simulink model "SchemaControlloDecentralizzatoSmartSixR2013a"  (Simulink 8.4)
settings: Solver=ode23  StartTime=0.0  StopTime=t(end)+Tf  FixedStep=T  RelTol=1e-3
PreLoadFcn:
  | initFunction
InitFcn:
  | initFunction
StopFcn:
  | figure
  | subplot(31,1)
  | plot(err_q.data(1:50))
  | subplot(312)
  | plot(err_dq.data(1:50))
  | subplot(313)
  | plot(err_ddq.data(1:50))
values from neighbouring files (symbols this model uses):
  FM = Kr^-1*Fv*Kr^-1    [ControlloreUnico.m]    (also in SimulazioneLsim.m = Kr^-1*Fv_att*Kr^-1; initFunction.m; initFunctionIm.m)
  Im = Kr^-1*Bconst*Kr^-1    [initFunction.m]    (also in initFunctionIm.m)
  KCA = diag([(-W(1,1)^2 + KM(1,1)*XR(1,1))/(KM(1,1)*KTA(1,1)*W(1,1)^2),             (-W(2,2)^2 + KM(2,2)*XR(2,2))/(KM(2,2)*KTA(2,2)*W(2,2)^2),             (-W(3,3)^2 + KM(3,3)*XR(3,3))/(KM(3,3)*KTA(3,3)*W(3,3)^2),             (-W(4,4)^2 + KM(4,4)*XR(4,4))/(KM(4,4)*KTA(4,4)*W(4,4)^2),             (-W(5,5)^2 + KM(5,5)*XR(5,5))/(KM(5,5)*KTA(5,5)*W(5,5)^2),             (-W(6,6)^2 + KM(6,6)*XR(6,6))/(KM(6,6)* ...(+20 chars)    [DesignControllersAcceleration_6.m]    (also in DesignControllersAcceleration_7.m; DiscreteControllersAcceleration_7.m)
  KCP = diag([(KTV(1,1)*W(1,1))/(2*KTP(1,1)*Z(1,1)),             (KTV(2,2)*W(2,2))/(2*KTP(2,2)*Z(2,2)),             (KTV(3,3)*W(3,3))/(2*KTP(3,3)*Z(3,3)),             (KTV(4,4)*W(4,4))/(2*KTP(4,4)*Z(4,4)),             (KTV(5,5)*W(5,5))/(2*KTP(5,5)*Z(5,5)),             (KTV(6,6)*W(6,6))/(2*KTP(6,6)*Z(6,6))])    [DesignControllersAcceleration_6.m]    (also in DesignControllersAcceleration_7.m; DesignControllersVelocity_6.m; DiscreteControllersAcceleration_7.m; DiscreteDesignControllersVelocity_6.m)
  KCV = diag([(2*KM(1,1)*KTA(1,1)*W(1,1)*XR(1,1)*Z(1,1))/(KTV(1,1)*(-W(1,1)^2 + KM(1,1)*XR(1,1))),             (2*KM(2,2)*KTA(2,2)*W(2,2)*XR(2,2)*Z(2,2))/(KTV(2,2)*(-W(2,2)^2 + KM(2,2)*XR(2,2))),             (2*KM(3,3)*KTA(3,3)*W(3,3)*XR(3,3)*Z(3,3))/(KTV(3,3)*(-W(3,3)^2 + KM(3,3)*XR(3,3))),             (2*KM(4,4)*KTA(4,4)*W(4,4)*XR(4,4)*Z(4,4))/(KTV(4,4)*(-W(4,4)^2 + KM(4,4)*XR(4,4))),             (2*KM( ...(+176 chars)    [DesignControllersAcceleration_6.m]    (also in DesignControllersAcceleration_7.m; DesignControllersVelocity_6.m = diag([(2*W(1,1)*Z(1,1))/(KM(1,1)*KTV(1,1)),             (2*W; DiscreteControllersAcceleration_7.m = diag([(rlkcv(1)*KM(1,1)*KTA(1,1)*W(1,1)*XR(1,1)*Z(1,1))/(KTV; DiscreteDesignControllersVelocity_6.m = diag([rlkcv(1)*(2*W(1,1)*Z(1,1))/(KM(1,1)*KTV(1,1)),        )
  KM = Kv^-1    [DesignControllersAcceleration_6.m]    (also in DesignControllersAcceleration_7.m; DesignControllersVelocity_6.m; DiscreteControllersAcceleration_7.m; DiscreteDesignControllersVelocity_6.m)
  KTA = diag([100 1 1 1 1 1])    [DesignControllersAcceleration_6.m]    (also in DesignControllersAcceleration_7.m = diag([1 1 1 1 1 1]); DiscreteControllersAcceleration_7.m = diag([1 1 1 1 1 1]))
  KTP = diag([9 1 1 1 1 1])    [DesignControllersAcceleration_6.m]    (also in DesignControllersAcceleration_7.m = diag([1 1 1 1 1 1]); DesignControllersVelocity_6.m = diag([1 1 1 1 1 1]); DiscreteControllersAcceleration_7.m = diag([1 1 1 1 1 1]); DiscreteDesignControllersVelocity_6.m = diag([1 1 1 1 1 1]))
  KTV = diag([4 1 1 1 1 1])    [DesignControllersAcceleration_6.m]    (also in DesignControllersAcceleration_7.m = diag([1 1 1 1 1 1]); DesignControllersVelocity_6.m = diag([1 1 1 1 1 1]); DiscreteControllersAcceleration_7.m = diag([1 1 1 1 1 1]); DiscreteDesignControllersVelocity_6.m = diag([1 1 1 1 1 1]))
  q0 = q0'    [initFunction.m]    (also in initFunctionIm.m)
  T = 0.05    [ComputeBconst_4.m]    (also in ControlloreUnico.m = 0.002; Identificazione_2.m = 0:1/F:(size(min_value,2)-1)*interval; Simulazione.m = 0.002; SimulazioneLsim.m = 0.002)
  TCA = diag([Tm(1,1) Tm(2,2) Tm(3,3) Tm(4,4) Tm(5,5) Tm(6,6)])    [DesignControllersAcceleration_6.m]    (also in DesignControllersAcceleration_7.m = diag([TM(1,1) TM(2,2) TM(3,3) TM(4,4) TM(5,5) TM(6,6)]); DiscreteControllersAcceleration_7.m = diag([TM(1,1) TM(2,2) TM(3,3) TM(4,4) TM(5,5) TM(6,6)]))
undefined symbols (not defined in the file or in its folder): Kr, Kt, Kv, La, Ra
libraries: simulink x18
(part 1 of 2)
CloseFcn:
  | rtwprivate ssgencode ModelCloseRequest ContributiCoppieComau
settings Model: Creator=Alessandro  LastModifiedBy=Leonardo  SimulationMode=accelerator  ExtModeAutoUpdateStatusClock=off  BufferReuse=off
settings DataIOCC: SaveFormat=StructureWithTime  SignalLoggingSaveFormat=Dataset
settings OptimizationCC: BlockReduction=off  BufferReuse=off  InitFltsAndDblsToZero=on
settings DebuggingCC: AlgebraicLoopMsg=none  SaveWithParameterizedLinksMsg=none  SignalResolutionControl=TryResolveAllWithWarning  SolverPrmCheckMsg=none  InheritedTsInSrcMsg=none  MultiTaskDSMMsg=warning  MultiTaskCondExecSysMsg=none  TasksWithSamePriorityMsg=none  UnconnectedInputMsg=none  UnconnectedOutputMsg=none  UnconnectedLineMsg=none  FrameProcessingCompatibilityMsg=error
settings GRTTargetCC: TargetFcnLib=ansi_tfl_tmw.mat
settings ConfigComp: CovMetricSettings=dw  CovHtmlReporting=on  CovSaveCumulativeToWorkspaceVar=on  CovSaveSingleToWorkspaceVar=on  CovModelRefEnable=Off  CovExternalEMLEnable=off

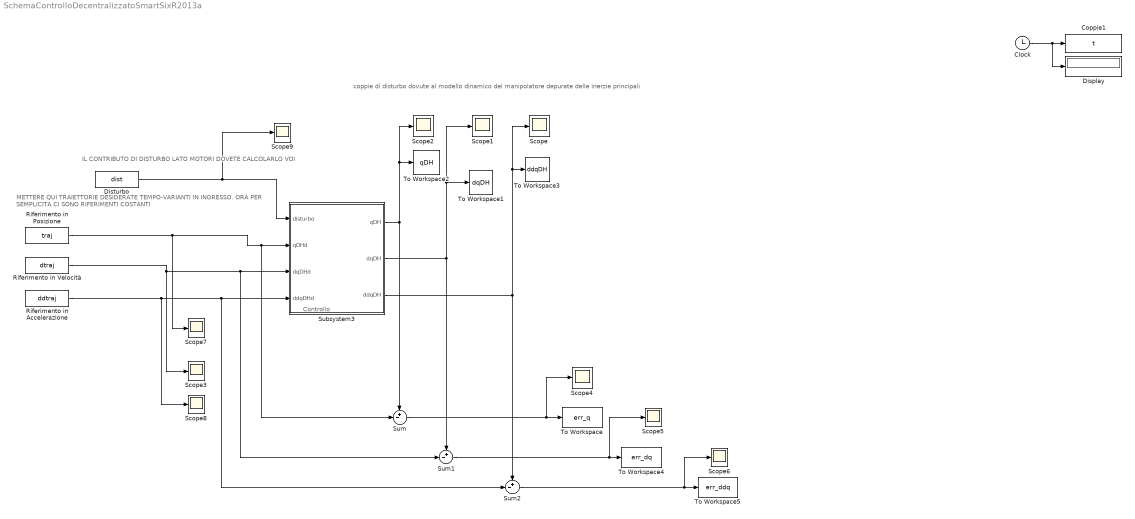
== system SchemaControlloDecentralizzatoSmartSixR2013a ==
  note: coppie di disturbo dovute al modello dinamico del manipolatore depurate delle inerzie principali
  note: Controllo
  note: METTERE QUI TRAIETTORIE DESIDERATE TEMPO-VARIANTI IN INGRESSO.
      | ORA PER SEMPLICITA CI SONO RIFERIMENTI COSTANTI
  note: IL CONTRIBUTO DI DISTURBO LATO MOTORI DOVETE CALCOLARLO VOI
  Clock : Clock
  Coppie1 : ToWorkspace  VariableName=t  SampleTime=-1
  Display : Display
  Disturbo : FromWorkspace  VariableName=dist  Interpolate=off  OutputAfterFinalValue=Holding final value
  Riferimento in Accelerazione : FromWorkspace  VariableName=ddtraj
  Riferimento in Posizione : FromWorkspace  VariableName=traj
  Riferimento in Velocità : FromWorkspace  VariableName=dtraj
  Scope{,1..9} (10 alike) : Scope
      Scope settings: TimeRange=0.4  YMin=-3427537178483172600000000000000000000000000000000000000000000000000000000000000000000000000000000000000000000000000000000000000000000000000000000000000000000000000000000000000000000000000000000000000000000000000000000000000000000000000000000000000000000000000000000000000000000000000000000000000000000.00000  YMax=6302006154523578300000000000000000000000000000000000000000000000000000000000000000000000000000000000000000000000000000000000000000000000000000000000000000000000000000000000000000000000000000000000000000000000000000000000000000000000000000000000000000000000000000000000000000000000000000000000000000000.00000
      Scope1 settings: YMin=-1.00000  YMax=1.00000
      Scope2 settings: TimeRange=0.01894736842105263  YMin=-1  YMax=1  SaveName=ScopeData2
      Scope3 settings: TimeRange=0.01894736842105263  YMin=-11.17185  YMax=11.83001  SaveName=ScopeData4
      Scope4 settings: TimeRange=5.918947368421053  YMin=-0.04  YMax=0.01
      Scope5 settings: TimeRange=5.018947368421053  YMin=-0.05  YMax=0.04  SaveName=ScopeData3
      Scope6 settings: TimeRange=1.018947368421053  YMin=-8  YMax=10  SaveName=ScopeData6
      Scope7 settings: TimeRange=0.01894736842105263  YMin=-1  YMax=1  SaveName=ScopeData2
      Scope8 settings: TimeRange=0.01894736842105263  YMin=-11.17185  YMax=11.83001  SaveName=ScopeData5
      Scope9 settings: TimeRange=0.01894736842105263  YMin=-1  YMax=1  SaveName=ScopeData7
  Subsystem3 : Subsystem
      mask Display:
      | disp('Controllo');
      | port_label('input', 1, 'disturbo');
      | port_label('input', 2, 'qDHd');
      | port_label('input', 3, 'dqDHd');
      | port_label('output', 1, 'qDH');
      | port_label('output', 2, 'dqDH');
      | port_label('output', 3, 'ddqDH');
  Sum : Sum  Inputs=+-|
  Sum1 : Sum  Inputs=+-|
  Sum2 : Sum  Inputs=+-|
  To Workspace : ToWorkspace  VariableName=err_q  SaveFormat=Timeseries  SampleTime=-1
  To Workspace1 : ToWorkspace  VariableName=dqDH  SampleTime=-1
  To Workspace2 : ToWorkspace  VariableName=qDH  SampleTime=-1
  To Workspace3 : ToWorkspace  VariableName=ddqDH  SampleTime=-1
  To Workspace4 : ToWorkspace  VariableName=err_dq  SaveFormat=Timeseries  SampleTime=-1
  To Workspace5 : ToWorkspace  VariableName=err_ddq  SaveFormat=Timeseries  SampleTime=-1
  wires:
  Clock/1 -> Coppie1/1, Display/1
  Subsystem3/2(dqDH) -> Sum1/1, To Workspace1/1, Scope1/1
  Subsystem3/1(qDH) -> To Workspace2/1, Scope2/1, Sum/1
  Subsystem3/3(ddqDH) -> Sum2/1, To Workspace3/1, Scope/1
  Riferimento in Velocità/1 -> Scope3/1, Sum1/2, Subsystem3/3(dqDHd)
  Riferimento in Accelerazione/1 -> Scope8/1, Sum2/2, Subsystem3/4(ddqDHd)
  Riferimento in Posizione/1 -> Scope7/1, Sum/2, Subsystem3/2(qDHd)
  Disturbo/1 -> Scope9/1, Subsystem3/1(disturbo)
  Sum/1 -> Scope4/1, To Workspace/1
  Sum1/1 -> Scope5/1, To Workspace4/1
  Sum2/1 -> Scope6/1, To Workspace5/1

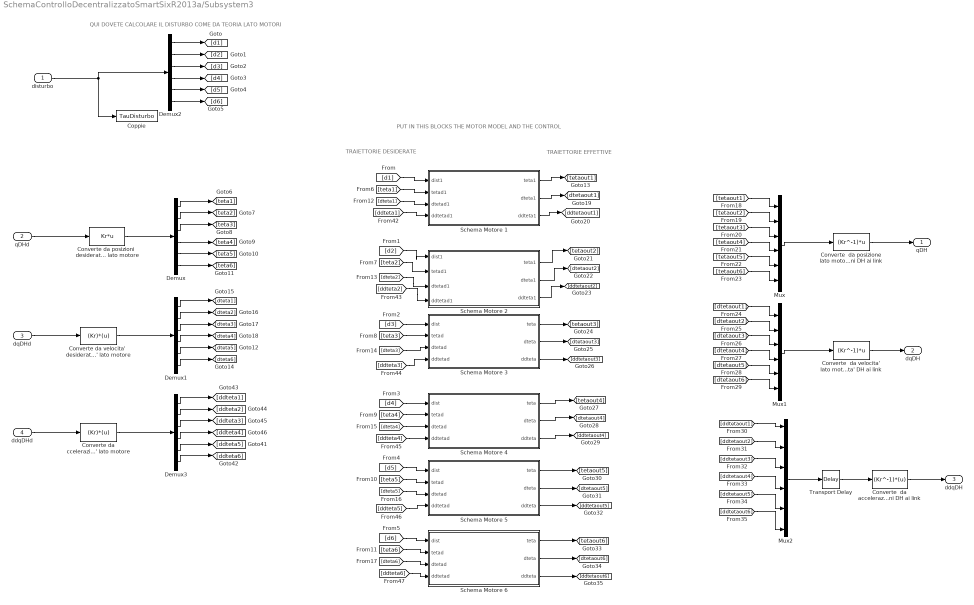
== system SchemaControlloDecentralizzatoSmartSixR2013a/Subsystem3 ==
  note: PUT IN THIS BLOCKS THE MOTOR MODEL AND THE CONTROL
  note: TRAIETTORIE DESIDERATE
  note: TRAIETTORIE EFFETTIVE
  note: QUI DOVETE CALCOLARE IL DISTURBO COME DA TEORIA LATO MOTORI
  disturbo : Inport
  qDHd : Inport  Port=2
  dqDHd : Inport  Port=3
  ddqDHd : Inport  Port=4
  Converte  da accelerazioni lato motore  ad accelerazioni DH ai link : MATLABFcn  MATLABFcn=(Kr^-1)*(u)
  "Converte  da posizione lato motore a  posizioni DH ai link " : MATLABFcn  MATLABFcn=(Kr^-1)*u
  "Converte  da velocita' lato motore  a velocita' DH ai link " : MATLABFcn  MATLABFcn=(Kr^-1)*u
  Converte da ccelerazioni  desiderate DH ai link  in velocita' lato motore : MATLABFcn  MATLABFcn=(Kr)*(u)
  "Converte da posizioni  desiderate DH ai link  in posizione lato motore " : MATLABFcn  MATLABFcn=Kr*u
  "Converte da velocita'  desiderate DH ai link  in velocita' lato motore " : MATLABFcn  MATLABFcn=(Kr)*(u)
  Coppie : ToWorkspace  VariableName=TauDisturbo  SampleTime=-1
  Demux{,1..3} (4 alike) : Demux  Outputs=6
  Mux : Mux  Inputs=6
  Mux1 : Mux  Inputs=6
  Mux2 : Mux  Inputs=6
  Schema Motore 1 : Subsystem  mask{i=1}
  Schema Motore 2 : Subsystem  mask{i=2}
  Schema Motore 3 : Subsystem  mask{i=3}
  Schema Motore 4 : Subsystem  mask{i=4}
  Schema Motore 5 : Subsystem  mask{i=5}
  Schema Motore 6 : Subsystem  mask{i=6}
  Transport Delay : TransportDelay  DelayTime=T
  qDH : Outport
  dqDH : Outport  Port=2
  ddqDH : Outport  Port=3
  wires:
  qDHd/1 -> "Converte da posizioni  desiderate DH ai link  in posizione lato motore "/1
  dqDHd/1 -> "Converte da velocita'  desiderate DH ai link  in velocita' lato motore "/1
  "Converte  da velocita' lato motore  a velocita' DH ai link "/1 -> dqDH/1
  Converte  da accelerazioni lato motore  ad accelerazioni DH ai link/1 -> ddqDH/1
  "Converte da posizioni  desiderate DH ai link  in posizione lato motore "/1 -> Demux/1
  disturbo/1 -> Coppie/1, Demux2/1
  "Converte  da posizione lato motore a  posizioni DH ai link "/1 -> qDH/1
  Mux/1 -> "Converte  da posizione lato motore a  posizioni DH ai link "/1
  Demux2/1 -> [d1]
  Demux2/2 -> [d2]
  Demux2/3 -> [d3]
  Demux2/4 -> [d4]
  Demux2/5 -> [d5]
  Demux2/6 -> [d6]
  [d3] -> Schema Motore 3/1(dist)
  Demux/1 -> [teta1]
  Demux/2 -> [teta2]
  Demux/3 -> [teta3]
  Demux/4 -> [teta4]
  Demux/5 -> [teta5]
  Demux/6 -> [teta6]
  [teta3] -> Schema Motore 3/2(tetad)
  "Converte da velocita'  desiderate DH ai link  in velocita' lato motore "/1 -> Demux1/1
  Demux1/1 -> [dteta1]
  Demux1/2 -> [dteta2]
  Demux1/3 -> [dteta3]
  Demux1/4 -> [dteta4]
  Demux1/5 -> [dteta5]
  Demux1/6 -> [dteta6]
  [dteta3] -> Schema Motore 3/3(dtetad)
  [tetaout1] -> Mux/1
  [tetaout2] -> Mux/2
  [tetaout3] -> Mux/3
  [tetaout4] -> Mux/4
  [tetaout5] -> Mux/5
  [tetaout6] -> Mux/6
  Mux1/1 -> "Converte  da velocita' lato motore  a velocita' DH ai link "/1
  [dtetaout1] -> Mux1/1
  [dtetaout2] -> Mux1/2
  [dtetaout3] -> Mux1/3
  [dtetaout4] -> Mux1/4
  [dtetaout5] -> Mux1/5
  [dtetaout6] -> Mux1/6
  [ddtetaout1] -> Mux2/1
  [ddtetaout2] -> Mux2/2
  [ddtetaout3] -> Mux2/3
  [ddtetaout4] -> Mux2/4
  [ddtetaout5] -> Mux2/5
  [ddtetaout6] -> Mux2/6
  ddqDHd/1 -> Converte da ccelerazioni  desiderate DH ai link  in velocita' lato motore/1
  Demux3/1 -> [ddteta1]
  Demux3/2 -> [ddteta2]
  Demux3/3 -> [ddteta3]
  Demux3/4 -> [ddteta4]
  Demux3/5 -> [ddteta5]
  Demux3/6 -> [ddteta6]
  Converte da ccelerazioni  desiderate DH ai link  in velocita' lato motore/1 -> Demux3/1
  Schema Motore 3/1(teta) -> [tetaout3]
  Schema Motore 3/2(dteta) -> [dtetaout3]
  Schema Motore 3/3(ddteta) -> [ddtetaout3]
  [ddteta3] -> Schema Motore 3/4(ddtetad)
  [d2] -> Schema Motore 2/1(dist1)
  [teta2] -> Schema Motore 2/2(tetad1)
  [dteta2] -> Schema Motore 2/3(dtetad1)
  [ddteta2] -> Schema Motore 2/4(ddtetad1)
  Schema Motore 2/1(teta1) -> [tetaout2]
  Schema Motore 2/2(dteta1) -> [dtetaout2]
  Schema Motore 2/3(ddteta1) -> [ddtetaout2]
  Mux2/1 -> Transport Delay/1
  Transport Delay/1 -> Converte  da accelerazioni lato motore  ad accelerazioni DH ai link/1
  [teta1] -> Schema Motore 1/2(tetad1)
  [dteta1] -> Schema Motore 1/3(dtetad1)
  [ddteta1] -> Schema Motore 1/4(ddtetad1)
  Schema Motore 1/1(teta1) -> [tetaout1]
  Schema Motore 1/2(dteta1) -> [dtetaout1]
  Schema Motore 1/3(ddteta1) -> [ddtetaout1]
  [d4] -> Schema Motore 4/1(dist)
  [teta4] -> Schema Motore 4/2(tetad)
  [dteta4] -> Schema Motore 4/3(dtetad)
  [ddteta4] -> Schema Motore 4/4(ddtetad)
  Schema Motore 4/1(teta) -> [tetaout4]
  Schema Motore 4/2(dteta) -> [dtetaout4]
  Schema Motore 4/3(ddteta) -> [ddtetaout4]
  [d5] -> Schema Motore 5/1(dist)
  [teta5] -> Schema Motore 5/2(tetad)
  [dteta5] -> Schema Motore 5/3(dtetad)
  [ddteta5] -> Schema Motore 5/4(ddtetad)
  [d6] -> Schema Motore 6/1(dist)
  [teta6] -> Schema Motore 6/2(tetad)
  [dteta6] -> Schema Motore 6/3(dtetad)
  [ddteta6] -> Schema Motore 6/4(ddtetad)
  Schema Motore 6/1(teta) -> [tetaout6]
  Schema Motore 6/2(dteta) -> [dtetaout6]
  Schema Motore 6/3(ddteta) -> [ddtetaout6]
  Schema Motore 5/3(ddteta) -> [ddtetaout5]
  Schema Motore 5/2(dteta) -> [dtetaout5]
  Schema Motore 5/1(teta) -> [tetaout5]
  [d1] -> Schema Motore 1/1(dist1)

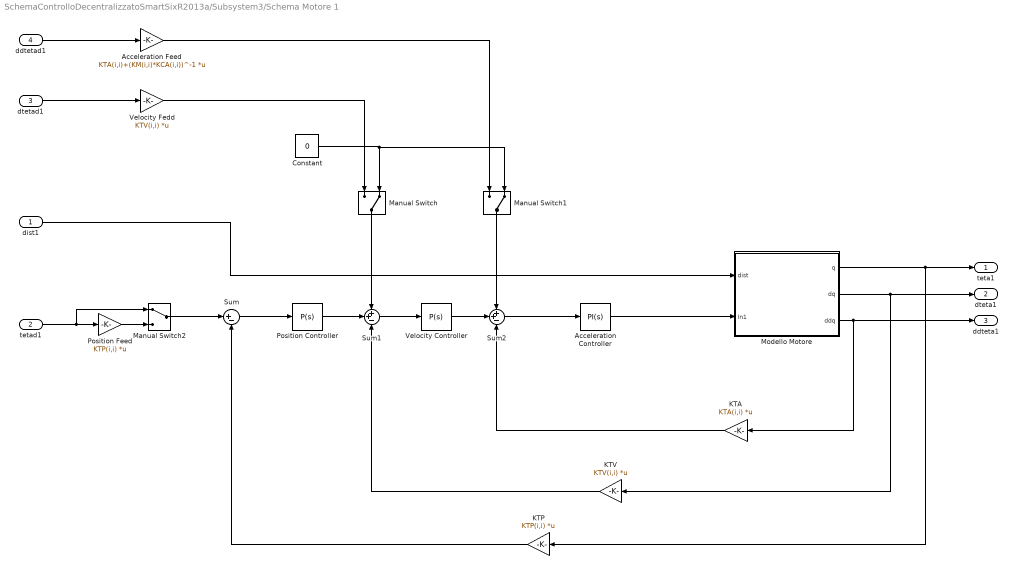
== system SchemaControlloDecentralizzatoSmartSixR2013a/Subsystem3/Schema Motore 1 ==
  dist1 : Inport  PortDimensions=1
  tetad1 : Inport  Port=2  PortDimensions=1
  dtetad1 : Inport  Port=3  PortDimensions=1
  ddtetad1 : Inport  Port=4  PortDimensions=1
  Acceleration Controller : simulink/Continuous/PID Controller  Controller=PI  TimeDomain=Continuous-time  SampleTime=-1  IntegratorMethod=Forward Euler  FilterMethod=Forward Euler  Form=Parallel  P=TCA(i,i)*KCA(i,i)  I=KCA(i,i)  D=0  N=100  InitialConditionSource=internal  InitialConditionForIntegrator=0  InitialConditionForFilter=0  ExternalReset=none  LimitOutput=off  UpperSaturationLimit=inf  LowerSaturationLimit=-inf  LinearizeAsGain=on  AntiWindupMode=none  Kb=1  TrackingMode=off  Kt=1  PParamMin=[]  PParamMax=[]  IParamMin=[]  IParamMax=[]  DParamMin=[]  DParamMax=[]  NParamMin=[]  NParamMax=[]  KbParamMin=[]  KbParamMax=[]  KtParamMin=[]  KtParamMax=[]  POutMin=[]  POutMax=[]  IOutMin=[]  IOutMax=[]  DOutMin=[]  DOutMax=[]  NOutMin=[]  NOutMax=[]  KbOutMin=[]  KbOutMax=[]  KtOutMin=[]  KtOutMax=[]  IntegratorOutMin=[]  IntegratorOutMax=[]  FilterOutMin=[]  FilterOutMax=[]  SumOutMin=[]  SumOutMax=[]  SumI1OutMin=[]  SumI1OutMax=[]  SumI2OutMin=[]  SumI2OutMax=[]  SumI3OutMin=[]  SumI3OutMax=[]  SumDOutMin=[]  SumDOutMax=[]  SaturationOutMin=[]  SaturationOutMax=[]  IntegratorContinuousStateAttributes=''  IntegratorStateMustResolveToSignalObject=off  IntegratorRTWStateStorageClass=Auto  FilterContinuousStateAttributes=''  FilterStateMustResolveToSignalObject=off  FilterRTWStateStorageClass=Auto  DifferentiatorICPrevScaledInput=0  DifferentiatorOutMin=[]  DifferentiatorOutMax=[]  UseFilter=on
  Acceleration Feed : Gain  Gain=KTA(i,i)+(KM(i,i)*KCA(i,i))^-1  Multiplication=Matrix(K*u)
  Constant : Constant  Value=0
  KTA : Gain  Gain=KTA(i,i)  Multiplication=Matrix(K*u)
  KTP : Gain  Gain=KTP(i,i)  Multiplication=Matrix(K*u)
  KTV : Gain  Gain=KTV(i,i)  Multiplication=Matrix(K*u)
  Manual Switch : ManualSwitch  CurrentSetting=0
  Manual Switch1 : ManualSwitch  CurrentSetting=0
  Manual Switch2 : ManualSwitch
  Modello Motore : Subsystem
  Position Controller : simulink/Continuous/PID Controller  Controller=P  TimeDomain=Continuous-time  SampleTime=-1  IntegratorMethod=Forward Euler  FilterMethod=Forward Euler  Form=Parallel  P=KCP(i,i)  I=1  D=0  N=100  InitialConditionSource=internal  InitialConditionForIntegrator=0  InitialConditionForFilter=0  ExternalReset=none  LimitOutput=off  UpperSaturationLimit=inf  LowerSaturationLimit=-inf  LinearizeAsGain=on  AntiWindupMode=none  Kb=1  TrackingMode=off  Kt=1  PParamMin=[]  PParamMax=[]  IParamMin=[]  IParamMax=[]  DParamMin=[]  DParamMax=[]  NParamMin=[]  NParamMax=[]  KbParamMin=[]  KbParamMax=[]  KtParamMin=[]  KtParamMax=[]  POutMin=[]  POutMax=[]  IOutMin=[]  IOutMax=[]  DOutMin=[]  DOutMax=[]  NOutMin=[]  NOutMax=[]  KbOutMin=[]  KbOutMax=[]  KtOutMin=[]  KtOutMax=[]  IntegratorOutMin=[]  IntegratorOutMax=[]  FilterOutMin=[]  FilterOutMax=[]  SumOutMin=[]  SumOutMax=[]  SumI1OutMin=[]  SumI1OutMax=[]  SumI2OutMin=[]  SumI2OutMax=[]  SumI3OutMin=[]  SumI3OutMax=[]  SumDOutMin=[]  SumDOutMax=[]  SaturationOutMin=[]  SaturationOutMax=[]  IntegratorContinuousStateAttributes=''  IntegratorStateMustResolveToSignalObject=off  IntegratorRTWStateStorageClass=Auto  FilterContinuousStateAttributes=''  FilterStateMustResolveToSignalObject=off  FilterRTWStateStorageClass=Auto  DifferentiatorICPrevScaledInput=0  DifferentiatorOutMin=[]  DifferentiatorOutMax=[]  UseFilter=on
  Position Feed : Gain  Gain=KTP(i,i)  Multiplication=Matrix(K*u)
  Sum : Sum  Inputs=|+-
  Sum1 : Sum  Inputs=++-
  Sum2 : Sum  Inputs=++-
  Velocity Controller : simulink/Continuous/PID Controller  Controller=P  TimeDomain=Continuous-time  SampleTime=-1  IntegratorMethod=Forward Euler  FilterMethod=Forward Euler  Form=Parallel  P=KCV(i,i)  I=1  D=0  N=100  InitialConditionSource=internal  InitialConditionForIntegrator=0  InitialConditionForFilter=0  ExternalReset=none  LimitOutput=off  UpperSaturationLimit=inf  LowerSaturationLimit=-inf  LinearizeAsGain=on  AntiWindupMode=none  Kb=1  TrackingMode=off  Kt=1  PParamMin=[]  PParamMax=[]  IParamMin=[]  IParamMax=[]  DParamMin=[]  DParamMax=[]  NParamMin=[]  NParamMax=[]  KbParamMin=[]  KbParamMax=[]  KtParamMin=[]  KtParamMax=[]  POutMin=[]  POutMax=[]  IOutMin=[]  IOutMax=[]  DOutMin=[]  DOutMax=[]  NOutMin=[]  NOutMax=[]  KbOutMin=[]  KbOutMax=[]  KtOutMin=[]  KtOutMax=[]  IntegratorOutMin=[]  IntegratorOutMax=[]  FilterOutMin=[]  FilterOutMax=[]  SumOutMin=[]  SumOutMax=[]  SumI1OutMin=[]  SumI1OutMax=[]  SumI2OutMin=[]  SumI2OutMax=[]  SumI3OutMin=[]  SumI3OutMax=[]  SumDOutMin=[]  SumDOutMax=[]  SaturationOutMin=[]  SaturationOutMax=[]  IntegratorContinuousStateAttributes=''  IntegratorStateMustResolveToSignalObject=off  IntegratorRTWStateStorageClass=Auto  FilterContinuousStateAttributes=''  FilterStateMustResolveToSignalObject=off  FilterRTWStateStorageClass=Auto  DifferentiatorICPrevScaledInput=0  DifferentiatorOutMin=[]  DifferentiatorOutMax=[]  UseFilter=on
  Velocity Fedd : Gain  Gain=KTV(i,i)  Multiplication=Matrix(K*u)
  teta1 : Outport  PortDimensions=1
  dteta1 : Outport  Port=2  PortDimensions=1
  ddteta1 : Outport  Port=3  PortDimensions=1
  wires:
  Sum/1 -> Position Controller/1
  Sum1/1 -> Velocity Controller/1
  Sum2/1 -> Acceleration Controller/1
  ddtetad1/1 -> Acceleration Feed/1
  KTP/1 -> Sum/2
  Acceleration Controller/1 -> Modello Motore/2(In1)
  dist1/1 -> Modello Motore/1(dist)
  Modello Motore/2(dq) -> dteta1/1, KTV/1
  Modello Motore/1(q) -> KTP/1, teta1/1
  Modello Motore/3(ddq) -> ddteta1/1, KTA/1
  Position Controller/1 -> Sum1/2
  KTV/1 -> Sum1/3
  Manual Switch/1 -> Sum1/1
  KTA/1 -> Sum2/3
  Velocity Controller/1 -> Sum2/2
  dtetad1/1 -> Velocity Fedd/1
  Constant/1 -> Manual Switch1/2, Manual Switch/2
  Manual Switch1/1 -> Sum2/1
  tetad1/1 -> Position Feed/1, Manual Switch2/1
  Manual Switch2/1 -> Sum/1
  Position Feed/1 -> Manual Switch2/2
  Velocity Fedd/1 -> Manual Switch/1
  Acceleration Feed/1 -> Manual Switch1/1

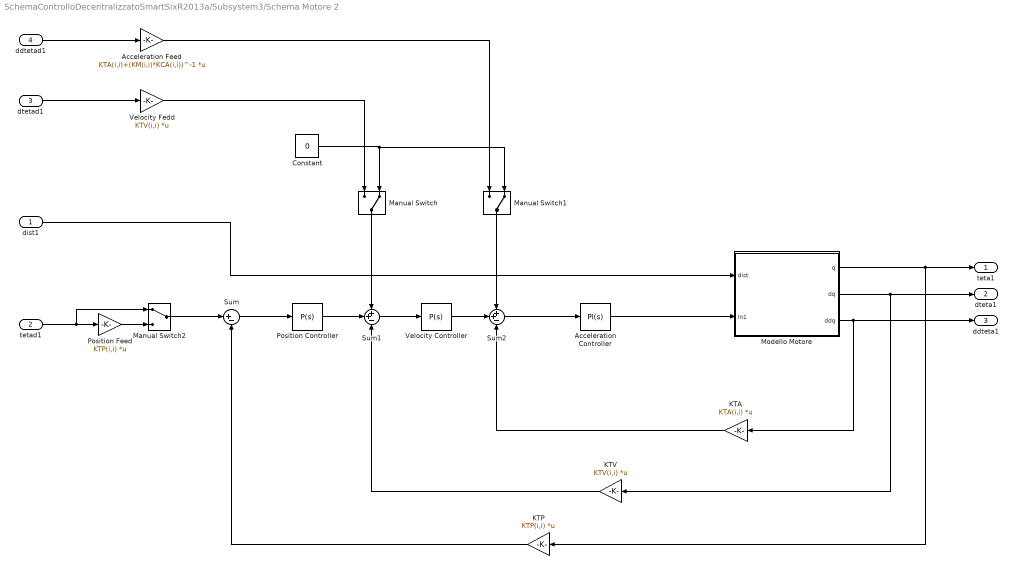
== system SchemaControlloDecentralizzatoSmartSixR2013a/Subsystem3/Schema Motore 2 ==
  dist1 : Inport  PortDimensions=1
  tetad1 : Inport  Port=2  PortDimensions=1
  dtetad1 : Inport  Port=3  PortDimensions=1
  ddtetad1 : Inport  Port=4  PortDimensions=1
  Acceleration Controller : simulink/Continuous/PID Controller  Controller=PI  TimeDomain=Continuous-time  SampleTime=-1  IntegratorMethod=Forward Euler  FilterMethod=Forward Euler  Form=Parallel  P=TCA(i,i)*KCA(i,i)  I=KCA(i,i)  D=0  N=100  InitialConditionSource=internal  InitialConditionForIntegrator=0  InitialConditionForFilter=0  ExternalReset=none  LimitOutput=off  UpperSaturationLimit=inf  LowerSaturationLimit=-inf  LinearizeAsGain=on  AntiWindupMode=none  Kb=1  TrackingMode=off  Kt=1  PParamMin=[]  PParamMax=[]  IParamMin=[]  IParamMax=[]  DParamMin=[]  DParamMax=[]  NParamMin=[]  NParamMax=[]  KbParamMin=[]  KbParamMax=[]  KtParamMin=[]  KtParamMax=[]  POutMin=[]  POutMax=[]  IOutMin=[]  IOutMax=[]  DOutMin=[]  DOutMax=[]  NOutMin=[]  NOutMax=[]  KbOutMin=[]  KbOutMax=[]  KtOutMin=[]  KtOutMax=[]  IntegratorOutMin=[]  IntegratorOutMax=[]  FilterOutMin=[]  FilterOutMax=[]  SumOutMin=[]  SumOutMax=[]  SumI1OutMin=[]  SumI1OutMax=[]  SumI2OutMin=[]  SumI2OutMax=[]  SumI3OutMin=[]  SumI3OutMax=[]  SumDOutMin=[]  SumDOutMax=[]  SaturationOutMin=[]  SaturationOutMax=[]  IntegratorContinuousStateAttributes=''  IntegratorStateMustResolveToSignalObject=off  IntegratorRTWStateStorageClass=Auto  FilterContinuousStateAttributes=''  FilterStateMustResolveToSignalObject=off  FilterRTWStateStorageClass=Auto  DifferentiatorICPrevScaledInput=0  DifferentiatorOutMin=[]  DifferentiatorOutMax=[]  UseFilter=on
  Acceleration Feed : Gain  Gain=KTA(i,i)+(KM(i,i)*KCA(i,i))^-1  Multiplication=Matrix(K*u)
  Constant : Constant  Value=0
  KTA : Gain  Gain=KTA(i,i)  Multiplication=Matrix(K*u)
  KTP : Gain  Gain=KTP(i,i)  Multiplication=Matrix(K*u)
  KTV : Gain  Gain=KTV(i,i)  Multiplication=Matrix(K*u)
  Manual Switch : ManualSwitch  CurrentSetting=0
  Manual Switch1 : ManualSwitch  CurrentSetting=0
  Manual Switch2 : ManualSwitch
  Modello Motore : Subsystem
  Position Controller : simulink/Continuous/PID Controller  Controller=P  TimeDomain=Continuous-time  SampleTime=-1  IntegratorMethod=Forward Euler  FilterMethod=Forward Euler  Form=Parallel  P=KCP(i,i)  I=1  D=0  N=100  InitialConditionSource=internal  InitialConditionForIntegrator=0  InitialConditionForFilter=0  ExternalReset=none  LimitOutput=off  UpperSaturationLimit=inf  LowerSaturationLimit=-inf  LinearizeAsGain=on  AntiWindupMode=none  Kb=1  TrackingMode=off  Kt=1  PParamMin=[]  PParamMax=[]  IParamMin=[]  IParamMax=[]  DParamMin=[]  DParamMax=[]  NParamMin=[]  NParamMax=[]  KbParamMin=[]  KbParamMax=[]  KtParamMin=[]  KtParamMax=[]  POutMin=[]  POutMax=[]  IOutMin=[]  IOutMax=[]  DOutMin=[]  DOutMax=[]  NOutMin=[]  NOutMax=[]  KbOutMin=[]  KbOutMax=[]  KtOutMin=[]  KtOutMax=[]  IntegratorOutMin=[]  IntegratorOutMax=[]  FilterOutMin=[]  FilterOutMax=[]  SumOutMin=[]  SumOutMax=[]  SumI1OutMin=[]  SumI1OutMax=[]  SumI2OutMin=[]  SumI2OutMax=[]  SumI3OutMin=[]  SumI3OutMax=[]  SumDOutMin=[]  SumDOutMax=[]  SaturationOutMin=[]  SaturationOutMax=[]  IntegratorContinuousStateAttributes=''  IntegratorStateMustResolveToSignalObject=off  IntegratorRTWStateStorageClass=Auto  FilterContinuousStateAttributes=''  FilterStateMustResolveToSignalObject=off  FilterRTWStateStorageClass=Auto  DifferentiatorICPrevScaledInput=0  DifferentiatorOutMin=[]  DifferentiatorOutMax=[]  UseFilter=on
  Position Feed : Gain  Gain=KTP(i,i)  Multiplication=Matrix(K*u)
  Sum : Sum  Inputs=|+-
  Sum1 : Sum  Inputs=++-
  Sum2 : Sum  Inputs=++-
  Velocity Controller : simulink/Continuous/PID Controller  Controller=P  TimeDomain=Continuous-time  SampleTime=-1  IntegratorMethod=Forward Euler  FilterMethod=Forward Euler  Form=Parallel  P=KCV(i,i)  I=1  D=0  N=100  InitialConditionSource=internal  InitialConditionForIntegrator=0  InitialConditionForFilter=0  ExternalReset=none  LimitOutput=off  UpperSaturationLimit=inf  LowerSaturationLimit=-inf  LinearizeAsGain=on  AntiWindupMode=none  Kb=1  TrackingMode=off  Kt=1  PParamMin=[]  PParamMax=[]  IParamMin=[]  IParamMax=[]  DParamMin=[]  DParamMax=[]  NParamMin=[]  NParamMax=[]  KbParamMin=[]  KbParamMax=[]  KtParamMin=[]  KtParamMax=[]  POutMin=[]  POutMax=[]  IOutMin=[]  IOutMax=[]  DOutMin=[]  DOutMax=[]  NOutMin=[]  NOutMax=[]  KbOutMin=[]  KbOutMax=[]  KtOutMin=[]  KtOutMax=[]  IntegratorOutMin=[]  IntegratorOutMax=[]  FilterOutMin=[]  FilterOutMax=[]  SumOutMin=[]  SumOutMax=[]  SumI1OutMin=[]  SumI1OutMax=[]  SumI2OutMin=[]  SumI2OutMax=[]  SumI3OutMin=[]  SumI3OutMax=[]  SumDOutMin=[]  SumDOutMax=[]  SaturationOutMin=[]  SaturationOutMax=[]  IntegratorContinuousStateAttributes=''  IntegratorStateMustResolveToSignalObject=off  IntegratorRTWStateStorageClass=Auto  FilterContinuousStateAttributes=''  FilterStateMustResolveToSignalObject=off  FilterRTWStateStorageClass=Auto  DifferentiatorICPrevScaledInput=0  DifferentiatorOutMin=[]  DifferentiatorOutMax=[]  UseFilter=on
  Velocity Fedd : Gain  Gain=KTV(i,i)  Multiplication=Matrix(K*u)
  teta1 : Outport  PortDimensions=1
  dteta1 : Outport  Port=2  PortDimensions=1
  ddteta1 : Outport  Port=3  PortDimensions=1
  wires:
  Sum/1 -> Position Controller/1
  Sum1/1 -> Velocity Controller/1
  Sum2/1 -> Acceleration Controller/1
  ddtetad1/1 -> Acceleration Feed/1
  KTP/1 -> Sum/2
  Acceleration Controller/1 -> Modello Motore/2(In1)
  dist1/1 -> Modello Motore/1(dist)
  Modello Motore/2(dq) -> dteta1/1, KTV/1
  Modello Motore/1(q) -> KTP/1, teta1/1
  Modello Motore/3(ddq) -> ddteta1/1, KTA/1
  Position Controller/1 -> Sum1/2
  KTV/1 -> Sum1/3
  Manual Switch/1 -> Sum1/1
  KTA/1 -> Sum2/3
  Velocity Controller/1 -> Sum2/2
  dtetad1/1 -> Velocity Fedd/1
  Constant/1 -> Manual Switch1/2, Manual Switch/2
  Manual Switch1/1 -> Sum2/1
  tetad1/1 -> Position Feed/1, Manual Switch2/1
  Manual Switch2/1 -> Sum/1
  Position Feed/1 -> Manual Switch2/2
  Velocity Fedd/1 -> Manual Switch/1
  Acceleration Feed/1 -> Manual Switch1/1

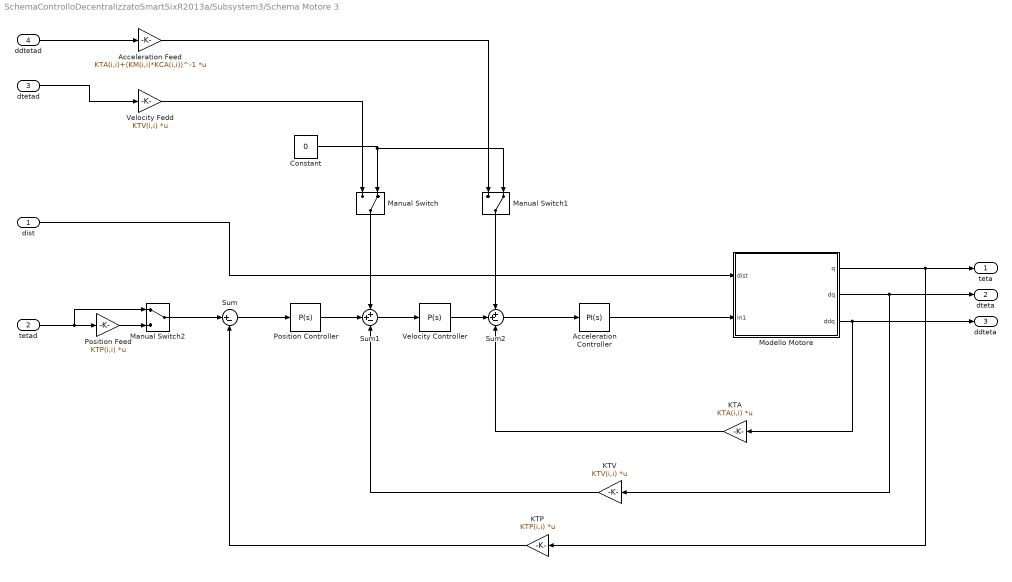
== system SchemaControlloDecentralizzatoSmartSixR2013a/Subsystem3/Schema Motore 3 ==
  dist : Inport  PortDimensions=1
  tetad : Inport  Port=2  PortDimensions=1
  dtetad : Inport  Port=3  PortDimensions=1
  ddtetad : Inport  Port=4  PortDimensions=1
  Acceleration Controller : simulink/Continuous/PID Controller  Controller=PI  TimeDomain=Continuous-time  SampleTime=-1  IntegratorMethod=Forward Euler  FilterMethod=Forward Euler  Form=Parallel  P=TCA(i,i)*KCA(i,i)  I=KCA(i,i)  D=0  N=100  InitialConditionSource=internal  InitialConditionForIntegrator=0  InitialConditionForFilter=0  ExternalReset=none  LimitOutput=off  UpperSaturationLimit=inf  LowerSaturationLimit=-inf  LinearizeAsGain=on  AntiWindupMode=none  Kb=1  TrackingMode=off  Kt=1  PParamMin=[]  PParamMax=[]  IParamMin=[]  IParamMax=[]  DParamMin=[]  DParamMax=[]  NParamMin=[]  NParamMax=[]  KbParamMin=[]  KbParamMax=[]  KtParamMin=[]  KtParamMax=[]  POutMin=[]  POutMax=[]  IOutMin=[]  IOutMax=[]  DOutMin=[]  DOutMax=[]  NOutMin=[]  NOutMax=[]  KbOutMin=[]  KbOutMax=[]  KtOutMin=[]  KtOutMax=[]  IntegratorOutMin=[]  IntegratorOutMax=[]  FilterOutMin=[]  FilterOutMax=[]  SumOutMin=[]  SumOutMax=[]  SumI1OutMin=[]  SumI1OutMax=[]  SumI2OutMin=[]  SumI2OutMax=[]  SumI3OutMin=[]  SumI3OutMax=[]  SumDOutMin=[]  SumDOutMax=[]  SaturationOutMin=[]  SaturationOutMax=[]  IntegratorContinuousStateAttributes=''  IntegratorStateMustResolveToSignalObject=off  IntegratorRTWStateStorageClass=Auto  FilterContinuousStateAttributes=''  FilterStateMustResolveToSignalObject=off  FilterRTWStateStorageClass=Auto  DifferentiatorICPrevScaledInput=0  DifferentiatorOutMin=[]  DifferentiatorOutMax=[]  UseFilter=on
  Acceleration Feed : Gain  Gain=KTA(i,i)+(KM(i,i)*KCA(i,i))^-1  Multiplication=Matrix(K*u)
  Constant : Constant  Value=0
  KTA : Gain  Gain=KTA(i,i)  Multiplication=Matrix(K*u)
  KTP : Gain  Gain=KTP(i,i)  Multiplication=Matrix(K*u)
  KTV : Gain  Gain=KTV(i,i)  Multiplication=Matrix(K*u)
  Manual Switch : ManualSwitch  CurrentSetting=0
  Manual Switch1 : ManualSwitch  CurrentSetting=0
  Manual Switch2 : ManualSwitch
  Modello Motore : Subsystem
  Position Controller : simulink/Continuous/PID Controller  Controller=P  TimeDomain=Continuous-time  SampleTime=-1  IntegratorMethod=Forward Euler  FilterMethod=Forward Euler  Form=Parallel  P=KCP(i,i)  I=1  D=0  N=100  InitialConditionSource=internal  InitialConditionForIntegrator=0  InitialConditionForFilter=0  ExternalReset=none  LimitOutput=off  UpperSaturationLimit=inf  LowerSaturationLimit=-inf  LinearizeAsGain=on  AntiWindupMode=none  Kb=1  TrackingMode=off  Kt=1  PParamMin=[]  PParamMax=[]  IParamMin=[]  IParamMax=[]  DParamMin=[]  DParamMax=[]  NParamMin=[]  NParamMax=[]  KbParamMin=[]  KbParamMax=[]  KtParamMin=[]  KtParamMax=[]  POutMin=[]  POutMax=[]  IOutMin=[]  IOutMax=[]  DOutMin=[]  DOutMax=[]  NOutMin=[]  NOutMax=[]  KbOutMin=[]  KbOutMax=[]  KtOutMin=[]  KtOutMax=[]  IntegratorOutMin=[]  IntegratorOutMax=[]  FilterOutMin=[]  FilterOutMax=[]  SumOutMin=[]  SumOutMax=[]  SumI1OutMin=[]  SumI1OutMax=[]  SumI2OutMin=[]  SumI2OutMax=[]  SumI3OutMin=[]  SumI3OutMax=[]  SumDOutMin=[]  SumDOutMax=[]  SaturationOutMin=[]  SaturationOutMax=[]  IntegratorContinuousStateAttributes=''  IntegratorStateMustResolveToSignalObject=off  IntegratorRTWStateStorageClass=Auto  FilterContinuousStateAttributes=''  FilterStateMustResolveToSignalObject=off  FilterRTWStateStorageClass=Auto  DifferentiatorICPrevScaledInput=0  DifferentiatorOutMin=[]  DifferentiatorOutMax=[]  UseFilter=on
  Position Feed : Gain  Gain=KTP(i,i)  Multiplication=Matrix(K*u)
  Sum : Sum  Inputs=|+-
  Sum1 : Sum  Inputs=++-
  Sum2 : Sum  Inputs=++-
  Velocity Controller : simulink/Continuous/PID Controller  Controller=P  TimeDomain=Continuous-time  SampleTime=-1  IntegratorMethod=Forward Euler  FilterMethod=Forward Euler  Form=Parallel  P=KCV(i,i)  I=1  D=0  N=100  InitialConditionSource=internal  InitialConditionForIntegrator=0  InitialConditionForFilter=0  ExternalReset=none  LimitOutput=off  UpperSaturationLimit=inf  LowerSaturationLimit=-inf  LinearizeAsGain=on  AntiWindupMode=none  Kb=1  TrackingMode=off  Kt=1  PParamMin=[]  PParamMax=[]  IParamMin=[]  IParamMax=[]  DParamMin=[]  DParamMax=[]  NParamMin=[]  NParamMax=[]  KbParamMin=[]  KbParamMax=[]  KtParamMin=[]  KtParamMax=[]  POutMin=[]  POutMax=[]  IOutMin=[]  IOutMax=[]  DOutMin=[]  DOutMax=[]  NOutMin=[]  NOutMax=[]  KbOutMin=[]  KbOutMax=[]  KtOutMin=[]  KtOutMax=[]  IntegratorOutMin=[]  IntegratorOutMax=[]  FilterOutMin=[]  FilterOutMax=[]  SumOutMin=[]  SumOutMax=[]  SumI1OutMin=[]  SumI1OutMax=[]  SumI2OutMin=[]  SumI2OutMax=[]  SumI3OutMin=[]  SumI3OutMax=[]  SumDOutMin=[]  SumDOutMax=[]  SaturationOutMin=[]  SaturationOutMax=[]  IntegratorContinuousStateAttributes=''  IntegratorStateMustResolveToSignalObject=off  IntegratorRTWStateStorageClass=Auto  FilterContinuousStateAttributes=''  FilterStateMustResolveToSignalObject=off  FilterRTWStateStorageClass=Auto  DifferentiatorICPrevScaledInput=0  DifferentiatorOutMin=[]  DifferentiatorOutMax=[]  UseFilter=on
  Velocity Fedd : Gain  Gain=KTV(i,i)  Multiplication=Matrix(K*u)
  teta : Outport  PortDimensions=1
  dteta : Outport  Port=2  PortDimensions=1
  ddteta : Outport  Port=3  PortDimensions=1
  wires:
  Sum/1 -> Position Controller/1
  Sum1/1 -> Velocity Controller/1
  Sum2/1 -> Acceleration Controller/1
  ddtetad/1 -> Acceleration Feed/1
  KTP/1 -> Sum/2
  Acceleration Controller/1 -> Modello Motore/2(In1)
  dist/1 -> Modello Motore/1(dist)
  Modello Motore/2(dq) -> dteta/1, KTV/1
  Modello Motore/1(q) -> teta/1, KTP/1
  Modello Motore/3(ddq) -> ddteta/1, KTA/1
  Position Controller/1 -> Sum1/2
  KTV/1 -> Sum1/3
  Manual Switch/1 -> Sum1/1
  KTA/1 -> Sum2/3
  Velocity Controller/1 -> Sum2/2
  Constant/1 -> Manual Switch1/2, Manual Switch/2
  Manual Switch1/1 -> Sum2/1
  tetad/1 -> Position Feed/1, Manual Switch2/1
  Manual Switch2/1 -> Sum/1
  Position Feed/1 -> Manual Switch2/2
  Velocity Fedd/1 -> Manual Switch/1
  Acceleration Feed/1 -> Manual Switch1/1
  dtetad/1 -> Velocity Fedd/1

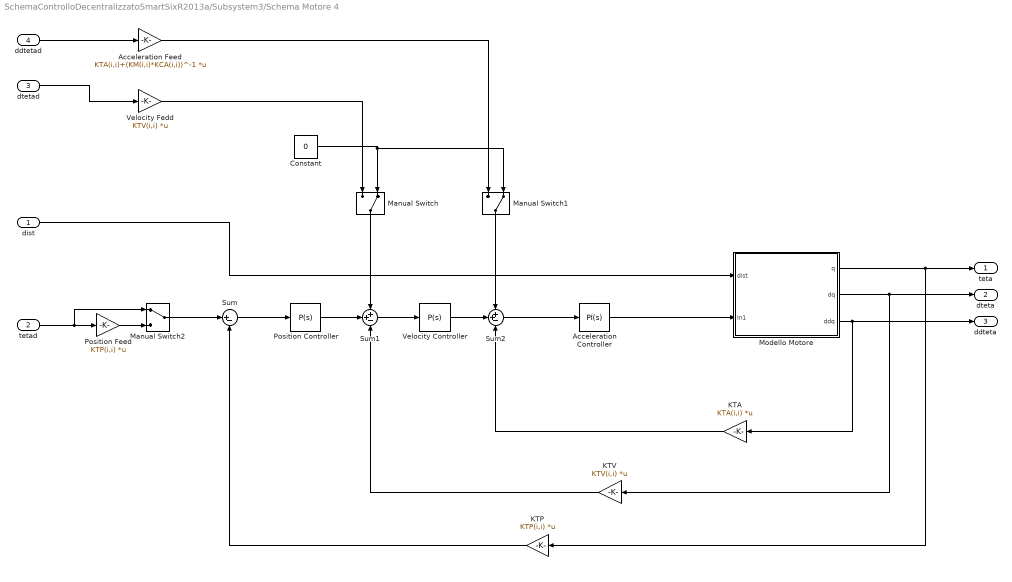
== system SchemaControlloDecentralizzatoSmartSixR2013a/Subsystem3/Schema Motore 4 ==
  dist : Inport  PortDimensions=1
  tetad : Inport  Port=2  PortDimensions=1
  dtetad : Inport  Port=3  PortDimensions=1
  ddtetad : Inport  Port=4  PortDimensions=1
  Acceleration Controller : simulink/Continuous/PID Controller  Controller=PI  TimeDomain=Continuous-time  SampleTime=-1  IntegratorMethod=Forward Euler  FilterMethod=Forward Euler  Form=Parallel  P=TCA(i,i)*KCA(i,i)  I=KCA(i,i)  D=0  N=100  InitialConditionSource=internal  InitialConditionForIntegrator=0  InitialConditionForFilter=0  ExternalReset=none  LimitOutput=off  UpperSaturationLimit=inf  LowerSaturationLimit=-inf  LinearizeAsGain=on  AntiWindupMode=none  Kb=1  TrackingMode=off  Kt=1  PParamMin=[]  PParamMax=[]  IParamMin=[]  IParamMax=[]  DParamMin=[]  DParamMax=[]  NParamMin=[]  NParamMax=[]  KbParamMin=[]  KbParamMax=[]  KtParamMin=[]  KtParamMax=[]  POutMin=[]  POutMax=[]  IOutMin=[]  IOutMax=[]  DOutMin=[]  DOutMax=[]  NOutMin=[]  NOutMax=[]  KbOutMin=[]  KbOutMax=[]  KtOutMin=[]  KtOutMax=[]  IntegratorOutMin=[]  IntegratorOutMax=[]  FilterOutMin=[]  FilterOutMax=[]  SumOutMin=[]  SumOutMax=[]  SumI1OutMin=[]  SumI1OutMax=[]  SumI2OutMin=[]  SumI2OutMax=[]  SumI3OutMin=[]  SumI3OutMax=[]  SumDOutMin=[]  SumDOutMax=[]  SaturationOutMin=[]  SaturationOutMax=[]  IntegratorContinuousStateAttributes=''  IntegratorStateMustResolveToSignalObject=off  IntegratorRTWStateStorageClass=Auto  FilterContinuousStateAttributes=''  FilterStateMustResolveToSignalObject=off  FilterRTWStateStorageClass=Auto  DifferentiatorICPrevScaledInput=0  DifferentiatorOutMin=[]  DifferentiatorOutMax=[]  UseFilter=on
  Acceleration Feed : Gain  Gain=KTA(i,i)+(KM(i,i)*KCA(i,i))^-1  Multiplication=Matrix(K*u)
  Constant : Constant  Value=0
  KTA : Gain  Gain=KTA(i,i)  Multiplication=Matrix(K*u)
  KTP : Gain  Gain=KTP(i,i)  Multiplication=Matrix(K*u)
  KTV : Gain  Gain=KTV(i,i)  Multiplication=Matrix(K*u)
  Manual Switch : ManualSwitch  CurrentSetting=0
  Manual Switch1 : ManualSwitch  CurrentSetting=0
  Manual Switch2 : ManualSwitch
  Modello Motore : Subsystem
  Position Controller : simulink/Continuous/PID Controller  Controller=P  TimeDomain=Continuous-time  SampleTime=-1  IntegratorMethod=Forward Euler  FilterMethod=Forward Euler  Form=Parallel  P=KCP(i,i)  I=1  D=0  N=100  InitialConditionSource=internal  InitialConditionForIntegrator=0  InitialConditionForFilter=0  ExternalReset=none  LimitOutput=off  UpperSaturationLimit=inf  LowerSaturationLimit=-inf  LinearizeAsGain=on  AntiWindupMode=none  Kb=1  TrackingMode=off  Kt=1  PParamMin=[]  PParamMax=[]  IParamMin=[]  IParamMax=[]  DParamMin=[]  DParamMax=[]  NParamMin=[]  NParamMax=[]  KbParamMin=[]  KbParamMax=[]  KtParamMin=[]  KtParamMax=[]  POutMin=[]  POutMax=[]  IOutMin=[]  IOutMax=[]  DOutMin=[]  DOutMax=[]  NOutMin=[]  NOutMax=[]  KbOutMin=[]  KbOutMax=[]  KtOutMin=[]  KtOutMax=[]  IntegratorOutMin=[]  IntegratorOutMax=[]  FilterOutMin=[]  FilterOutMax=[]  SumOutMin=[]  SumOutMax=[]  SumI1OutMin=[]  SumI1OutMax=[]  SumI2OutMin=[]  SumI2OutMax=[]  SumI3OutMin=[]  SumI3OutMax=[]  SumDOutMin=[]  SumDOutMax=[]  SaturationOutMin=[]  SaturationOutMax=[]  IntegratorContinuousStateAttributes=''  IntegratorStateMustResolveToSignalObject=off  IntegratorRTWStateStorageClass=Auto  FilterContinuousStateAttributes=''  FilterStateMustResolveToSignalObject=off  FilterRTWStateStorageClass=Auto  DifferentiatorICPrevScaledInput=0  DifferentiatorOutMin=[]  DifferentiatorOutMax=[]  UseFilter=on
  Position Feed : Gain  Gain=KTP(i,i)  Multiplication=Matrix(K*u)
  Sum : Sum  Inputs=|+-
  Sum1 : Sum  Inputs=++-
  Sum2 : Sum  Inputs=++-
  Velocity Controller : simulink/Continuous/PID Controller  Controller=P  TimeDomain=Continuous-time  SampleTime=-1  IntegratorMethod=Forward Euler  FilterMethod=Forward Euler  Form=Parallel  P=KCV(i,i)  I=1  D=0  N=100  InitialConditionSource=internal  InitialConditionForIntegrator=0  InitialConditionForFilter=0  ExternalReset=none  LimitOutput=off  UpperSaturationLimit=inf  LowerSaturationLimit=-inf  LinearizeAsGain=on  AntiWindupMode=none  Kb=1  TrackingMode=off  Kt=1  PParamMin=[]  PParamMax=[]  IParamMin=[]  IParamMax=[]  DParamMin=[]  DParamMax=[]  NParamMin=[]  NParamMax=[]  KbParamMin=[]  KbParamMax=[]  KtParamMin=[]  KtParamMax=[]  POutMin=[]  POutMax=[]  IOutMin=[]  IOutMax=[]  DOutMin=[]  DOutMax=[]  NOutMin=[]  NOutMax=[]  KbOutMin=[]  KbOutMax=[]  KtOutMin=[]  KtOutMax=[]  IntegratorOutMin=[]  IntegratorOutMax=[]  FilterOutMin=[]  FilterOutMax=[]  SumOutMin=[]  SumOutMax=[]  SumI1OutMin=[]  SumI1OutMax=[]  SumI2OutMin=[]  SumI2OutMax=[]  SumI3OutMin=[]  SumI3OutMax=[]  SumDOutMin=[]  SumDOutMax=[]  SaturationOutMin=[]  SaturationOutMax=[]  IntegratorContinuousStateAttributes=''  IntegratorStateMustResolveToSignalObject=off  IntegratorRTWStateStorageClass=Auto  FilterContinuousStateAttributes=''  FilterStateMustResolveToSignalObject=off  FilterRTWStateStorageClass=Auto  DifferentiatorICPrevScaledInput=0  DifferentiatorOutMin=[]  DifferentiatorOutMax=[]  UseFilter=on
  Velocity Fedd : Gain  Gain=KTV(i,i)  Multiplication=Matrix(K*u)
  teta : Outport  PortDimensions=1
  dteta : Outport  Port=2  PortDimensions=1
  ddteta : Outport  Port=3  PortDimensions=1
  wires:
  Sum/1 -> Position Controller/1
  Sum1/1 -> Velocity Controller/1
  Sum2/1 -> Acceleration Controller/1
  ddtetad/1 -> Acceleration Feed/1
  KTP/1 -> Sum/2
  Acceleration Controller/1 -> Modello Motore/2(In1)
  dist/1 -> Modello Motore/1(dist)
  Modello Motore/2(dq) -> dteta/1, KTV/1
  Modello Motore/1(q) -> teta/1, KTP/1
  Modello Motore/3(ddq) -> ddteta/1, KTA/1
  Position Controller/1 -> Sum1/2
  KTV/1 -> Sum1/3
  Manual Switch/1 -> Sum1/1
  KTA/1 -> Sum2/3
  Velocity Controller/1 -> Sum2/2
  Constant/1 -> Manual Switch1/2, Manual Switch/2
  Manual Switch1/1 -> Sum2/1
  tetad/1 -> Position Feed/1, Manual Switch2/1
  Manual Switch2/1 -> Sum/1
  Position Feed/1 -> Manual Switch2/2
  Velocity Fedd/1 -> Manual Switch/1
  Acceleration Feed/1 -> Manual Switch1/1
  dtetad/1 -> Velocity Fedd/1

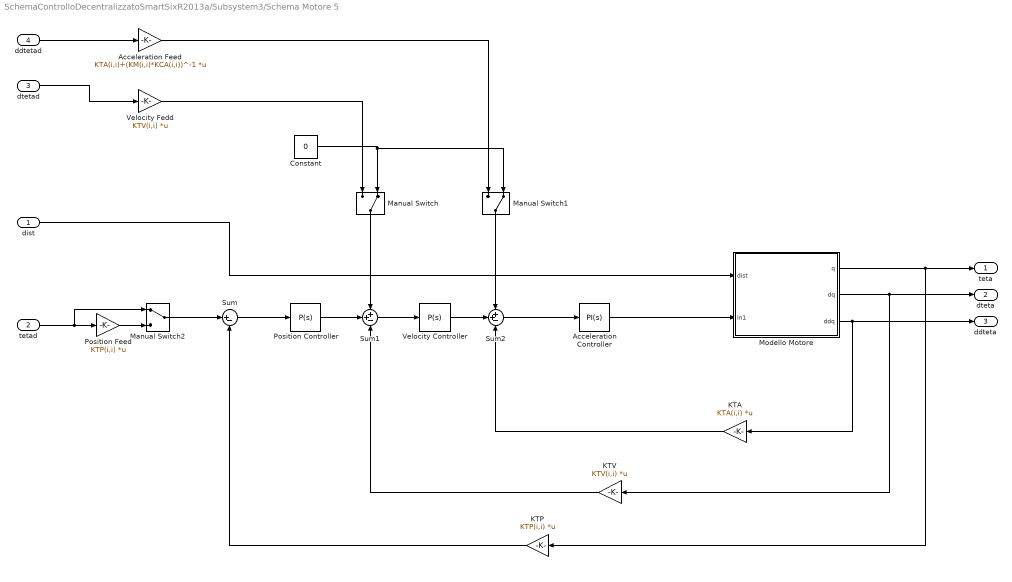
== system SchemaControlloDecentralizzatoSmartSixR2013a/Subsystem3/Schema Motore 5 ==
  dist : Inport  PortDimensions=1
  tetad : Inport  Port=2  PortDimensions=1
  dtetad : Inport  Port=3  PortDimensions=1
  ddtetad : Inport  Port=4  PortDimensions=1
  Acceleration Controller : simulink/Continuous/PID Controller  Controller=PI  TimeDomain=Continuous-time  SampleTime=-1  IntegratorMethod=Forward Euler  FilterMethod=Forward Euler  Form=Parallel  P=TCA(i,i)*KCA(i,i)  I=KCA(i,i)  D=0  N=100  InitialConditionSource=internal  InitialConditionForIntegrator=0  InitialConditionForFilter=0  ExternalReset=none  LimitOutput=off  UpperSaturationLimit=inf  LowerSaturationLimit=-inf  LinearizeAsGain=on  AntiWindupMode=none  Kb=1  TrackingMode=off  Kt=1  PParamMin=[]  PParamMax=[]  IParamMin=[]  IParamMax=[]  DParamMin=[]  DParamMax=[]  NParamMin=[]  NParamMax=[]  KbParamMin=[]  KbParamMax=[]  KtParamMin=[]  KtParamMax=[]  POutMin=[]  POutMax=[]  IOutMin=[]  IOutMax=[]  DOutMin=[]  DOutMax=[]  NOutMin=[]  NOutMax=[]  KbOutMin=[]  KbOutMax=[]  KtOutMin=[]  KtOutMax=[]  IntegratorOutMin=[]  IntegratorOutMax=[]  FilterOutMin=[]  FilterOutMax=[]  SumOutMin=[]  SumOutMax=[]  SumI1OutMin=[]  SumI1OutMax=[]  SumI2OutMin=[]  SumI2OutMax=[]  SumI3OutMin=[]  SumI3OutMax=[]  SumDOutMin=[]  SumDOutMax=[]  SaturationOutMin=[]  SaturationOutMax=[]  IntegratorContinuousStateAttributes=''  IntegratorStateMustResolveToSignalObject=off  IntegratorRTWStateStorageClass=Auto  FilterContinuousStateAttributes=''  FilterStateMustResolveToSignalObject=off  FilterRTWStateStorageClass=Auto  DifferentiatorICPrevScaledInput=0  DifferentiatorOutMin=[]  DifferentiatorOutMax=[]  UseFilter=on
  Acceleration Feed : Gain  Gain=KTA(i,i)+(KM(i,i)*KCA(i,i))^-1  Multiplication=Matrix(K*u)
  Constant : Constant  Value=0
  KTA : Gain  Gain=KTA(i,i)  Multiplication=Matrix(K*u)
  KTP : Gain  Gain=KTP(i,i)  Multiplication=Matrix(K*u)
  KTV : Gain  Gain=KTV(i,i)  Multiplication=Matrix(K*u)
  Manual Switch : ManualSwitch  CurrentSetting=0
  Manual Switch1 : ManualSwitch  CurrentSetting=0
  Manual Switch2 : ManualSwitch
  Modello Motore : Subsystem
  Position Controller : simulink/Continuous/PID Controller  Controller=P  TimeDomain=Continuous-time  SampleTime=-1  IntegratorMethod=Forward Euler  FilterMethod=Forward Euler  Form=Parallel  P=KCP(i,i)  I=1  D=0  N=100  InitialConditionSource=internal  InitialConditionForIntegrator=0  InitialConditionForFilter=0  ExternalReset=none  LimitOutput=off  UpperSaturationLimit=inf  LowerSaturationLimit=-inf  LinearizeAsGain=on  AntiWindupMode=none  Kb=1  TrackingMode=off  Kt=1  PParamMin=[]  PParamMax=[]  IParamMin=[]  IParamMax=[]  DParamMin=[]  DParamMax=[]  NParamMin=[]  NParamMax=[]  KbParamMin=[]  KbParamMax=[]  KtParamMin=[]  KtParamMax=[]  POutMin=[]  POutMax=[]  IOutMin=[]  IOutMax=[]  DOutMin=[]  DOutMax=[]  NOutMin=[]  NOutMax=[]  KbOutMin=[]  KbOutMax=[]  KtOutMin=[]  KtOutMax=[]  IntegratorOutMin=[]  IntegratorOutMax=[]  FilterOutMin=[]  FilterOutMax=[]  SumOutMin=[]  SumOutMax=[]  SumI1OutMin=[]  SumI1OutMax=[]  SumI2OutMin=[]  SumI2OutMax=[]  SumI3OutMin=[]  SumI3OutMax=[]  SumDOutMin=[]  SumDOutMax=[]  SaturationOutMin=[]  SaturationOutMax=[]  IntegratorContinuousStateAttributes=''  IntegratorStateMustResolveToSignalObject=off  IntegratorRTWStateStorageClass=Auto  FilterContinuousStateAttributes=''  FilterStateMustResolveToSignalObject=off  FilterRTWStateStorageClass=Auto  DifferentiatorICPrevScaledInput=0  DifferentiatorOutMin=[]  DifferentiatorOutMax=[]  UseFilter=on
  Position Feed : Gain  Gain=KTP(i,i)  Multiplication=Matrix(K*u)
  Sum : Sum  Inputs=|+-
  Sum1 : Sum  Inputs=++-
  Sum2 : Sum  Inputs=++-
  Velocity Controller : simulink/Continuous/PID Controller  Controller=P  TimeDomain=Continuous-time  SampleTime=-1  IntegratorMethod=Forward Euler  FilterMethod=Forward Euler  Form=Parallel  P=KCV(i,i)  I=1  D=0  N=100  InitialConditionSource=internal  InitialConditionForIntegrator=0  InitialConditionForFilter=0  ExternalReset=none  LimitOutput=off  UpperSaturationLimit=inf  LowerSaturationLimit=-inf  LinearizeAsGain=on  AntiWindupMode=none  Kb=1  TrackingMode=off  Kt=1  PParamMin=[]  PParamMax=[]  IParamMin=[]  IParamMax=[]  DParamMin=[]  DParamMax=[]  NParamMin=[]  NParamMax=[]  KbParamMin=[]  KbParamMax=[]  KtParamMin=[]  KtParamMax=[]  POutMin=[]  POutMax=[]  IOutMin=[]  IOutMax=[]  DOutMin=[]  DOutMax=[]  NOutMin=[]  NOutMax=[]  KbOutMin=[]  KbOutMax=[]  KtOutMin=[]  KtOutMax=[]  IntegratorOutMin=[]  IntegratorOutMax=[]  FilterOutMin=[]  FilterOutMax=[]  SumOutMin=[]  SumOutMax=[]  SumI1OutMin=[]  SumI1OutMax=[]  SumI2OutMin=[]  SumI2OutMax=[]  SumI3OutMin=[]  SumI3OutMax=[]  SumDOutMin=[]  SumDOutMax=[]  SaturationOutMin=[]  SaturationOutMax=[]  IntegratorContinuousStateAttributes=''  IntegratorStateMustResolveToSignalObject=off  IntegratorRTWStateStorageClass=Auto  FilterContinuousStateAttributes=''  FilterStateMustResolveToSignalObject=off  FilterRTWStateStorageClass=Auto  DifferentiatorICPrevScaledInput=0  DifferentiatorOutMin=[]  DifferentiatorOutMax=[]  UseFilter=on
  Velocity Fedd : Gain  Gain=KTV(i,i)  Multiplication=Matrix(K*u)
  teta : Outport  PortDimensions=1
  dteta : Outport  Port=2  PortDimensions=1
  ddteta : Outport  Port=3  PortDimensions=1
  wires:
  Sum/1 -> Position Controller/1
  Sum1/1 -> Velocity Controller/1
  Sum2/1 -> Acceleration Controller/1
  ddtetad/1 -> Acceleration Feed/1
  KTP/1 -> Sum/2
  Acceleration Controller/1 -> Modello Motore/2(In1)
  dist/1 -> Modello Motore/1(dist)
  Modello Motore/2(dq) -> dteta/1, KTV/1
  Modello Motore/1(q) -> teta/1, KTP/1
  Modello Motore/3(ddq) -> ddteta/1, KTA/1
  Position Controller/1 -> Sum1/2
  KTV/1 -> Sum1/3
  Manual Switch/1 -> Sum1/1
  KTA/1 -> Sum2/3
  Velocity Controller/1 -> Sum2/2
  Constant/1 -> Manual Switch1/2, Manual Switch/2
  Manual Switch1/1 -> Sum2/1
  tetad/1 -> Position Feed/1, Manual Switch2/1
  Manual Switch2/1 -> Sum/1
  Position Feed/1 -> Manual Switch2/2
  Velocity Fedd/1 -> Manual Switch/1
  Acceleration Feed/1 -> Manual Switch1/1
  dtetad/1 -> Velocity Fedd/1
